simulink model "Doble_pendulo"  (R2024a)
settings: Solver=VariableStepAuto  StartTime=0.0  StopTime=10.0  RelTol=1e-3
values from neighbouring files (symbols this model uses):
  g = 9.81    [exp1.m]
  l1 = 0.3    [exp1.m]
  l2 = 0.25    [exp1.m]
  m1 = 0.2    [exp1.m]
  m2 = 0.1    [exp1.m]
settings Model: Creator=Braulio Ramíreza  LastModifiedBy=Braulio Ramíreza

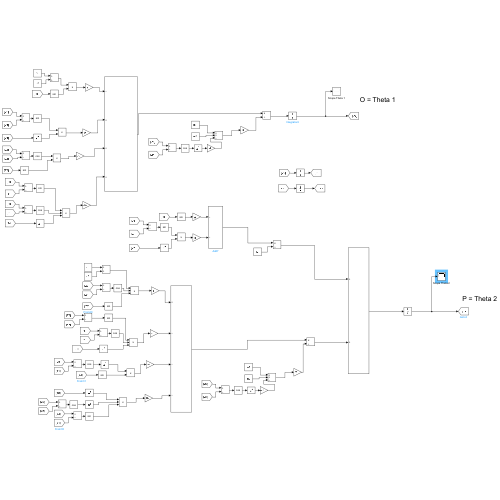
[thumbnail: Simulink's stored preview of the top-level diagram]
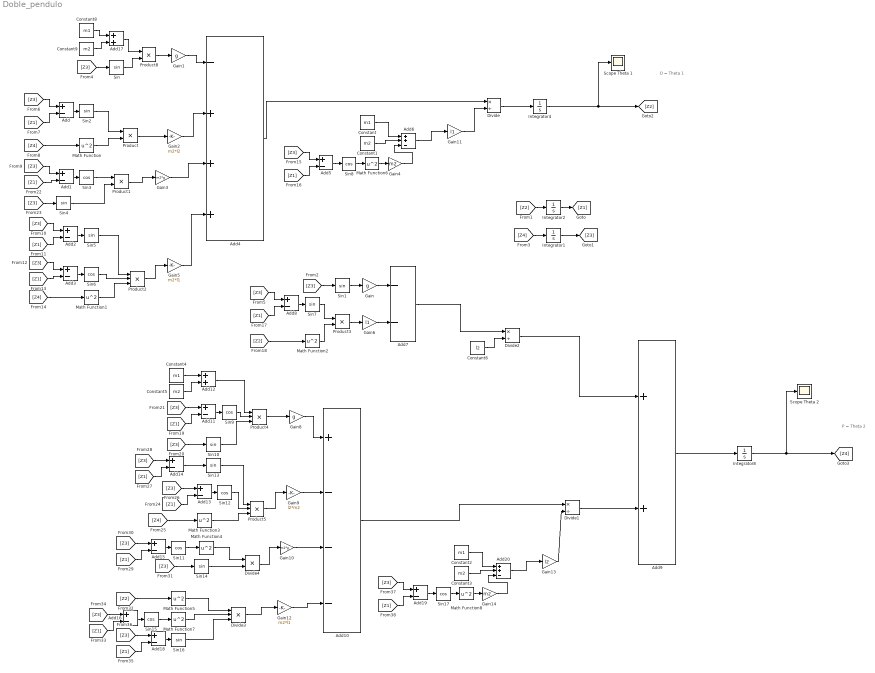
== system Doble_pendulo ==
  note: P = Theta 2
  note: O = Theta 1
  Add{,1..3,5,8,11,13..16,18..19} (13 alike) : Sum  Inputs=+-
  Add10 : Sum  Inputs=+---
  Add12 : Sum
  Add17 : Sum
  Add20 : Sum  Inputs=++-
  Add4 : Sum  Inputs=-+++
  Add6 : Sum  Inputs=++-
  Add7 : Sum  Inputs=--
  Add9 : Sum
  Constant{,2,4,8} (4 alike) : Constant  Value=m1
  Constant{1,3,5,9} (4 alike) : Constant  Value=m2
  Constant6 : Constant  Value=l2
  Divide : Product  Inputs=*/
  Divide1 : Product  Inputs=*/
  Divide2 : Product  Inputs=*/
  Divide3 : Product  Inputs=***
  Divide4 : Product  Inputs=**
  Gain : Gain  Gain=g
  Gain1 : Gain  Gain=g
  Gain10 : Gain  Gain=m2*g
  Gain11 : Gain  Gain=l1
  Gain12 : Gain  Gain=m2*l1
  Gain13 : Gain  Gain=l2
  Gain14 : Gain  Gain=m2
  Gain2 : Gain  Gain=m2*l2
  Gain3 : Gain  Gain=m2*g
  Gain4 : Gain  Gain=m2
  Gain5 : Gain  Gain=m2*l1
  Gain6 : Gain  Gain=l1
  Gain8 : Gain  Gain=g
  Gain9 : Gain  Gain=l2*m2
  Integrator1 : Integrator
  Integrator2 : Integrator
  Integrator4 : Integrator
  Integrator8 : Integrator  InitialCondition=(35*pi)/180
  Math Function{,1..8} (9 alike) : Math  Operator=square
  Product{,1,3,8} (4 alike) : Product
  Product2 : Product  Inputs=3
  Product4 : Product  Inputs=3
  Product5 : Product  Inputs=3
  Scope Theta 1 : Scope
  Scope Theta 2 : Scope
  Sin{,1..2,4..5,7,10,13..14,16} (10 alike) : Trigonometry
  Sin{3,6,8..9,11..12,15,17} (8 alike) : Trigonometry  Operator=cos
  wires:
  [Z2] -> Integrator2/1
  Integrator2/1 -> [Z1]
  Integrator1/1 -> [Z3]
  [Z4] -> Integrator1/1
  Sin15/1 -> Math Function7/1
  Constant4/1 -> Add12/1
  [Z1] -> Add15/2
  Sin/1 -> Product8/2
  Add19/1 -> Sin17/1
  Add13/1 -> Sin12/1
  Add10/1 -> Divide1/1
  Gain/1 -> Add7/1
  [Z1] -> Add3/2
  Math Function8/1 -> Gain14/1
  Constant3/1 -> Add20/2
  Divide3/1 -> Gain12/1
  Gain1/1 -> Add4/1
  [Z1] -> Add5/2
  [Z1] -> Add2/2
  Math Function4/1 -> Divide4/1
  Gain5/1 -> Add4/4
  Sin17/1 -> Math Function8/1
  Add20/1 -> Gain13/1
  [Z3] -> Add19/1
  [Z3] -> Add14/1
  Gain12/1 -> Add10/4
  Add2/1 -> Sin5/1
  Math Function5/1 -> Divide3/1
  Divide4/1 -> Gain10/1
  [Z2] -> Math Function5/1
  [Z3] -> Add15/1
  [Z3] -> Add16/1
  Add15/1 -> Sin11/1
  Product3/1 -> Gain6/1
  Add1/1 -> Sin3/1
  [Z3] -> Add/1
  Constant5/1 -> Add12/2
  Constant8/1 -> Add17/1
  Math Function3/1 -> Product5/3
  [Z1] -> Add18/2
  [Z1] -> Add/2
  Constant9/1 -> Add17/2
  [Z1] -> Add14/2
  Add12/1 -> Product4/1
  Add14/1 -> Sin13/1
  [Z1] -> Add8/2
  Divide/1 -> Integrator4/1
  [Z3] -> Add5/1
  Sin13/1 -> Product5/1
  Sin12/1 -> Product5/2
  [Z3] -> Sin10/1
  [Z3] -> Add13/1
  [Z1] -> Add13/2
  Sin9/1 -> Product4/2
  Gain2/1 -> Add4/2
  Sin11/1 -> Math Function4/1
  [Z3] -> Add11/1
  Add8/1 -> Sin7/1
  [Z3] -> Sin14/1
  [Z2] -> Math Function2/1
  Gain6/1 -> Add7/2
  Sin1/1 -> Gain/1
  Math Function2/1 -> Product3/2
  Add17/1 -> Product8/1
  Sin5/1 -> Product2/1
  Sin4/1 -> Product1/2
  Product8/1 -> Gain1/1
  Add11/1 -> Sin9/1
  Add/1 -> Sin2/1
  Math Function1/1 -> Product2/3
  Add3/1 -> Sin6/1
  Product5/1 -> Gain9/1
  Add6/1 -> Gain11/1
  Product2/1 -> Gain5/1
  Add4/1 -> Divide/1
  [Z1] -> Add11/2
  [Z4] -> Math Function1/1
  Sin8/1 -> Math Function6/1
  Gain4/1 -> Add6/3
  [Z3] -> Add3/1
  [Z3] -> Add2/1
  Math Function6/1 -> Gain4/1
  [Z1] -> Add1/2
  Sin2/1 -> Product/1
  Gain3/1 -> Add4/3
  Product1/1 -> Gain3/1
  Math Function/1 -> Product/2
  Product/1 -> Gain2/1
  [Z3] -> Sin/1
  Add9/1 -> Integrator8/1
  Constant1/1 -> Add6/2
  [Z3] -> Add8/1
  Sin16/1 -> Divide3/3
  [Z3] -> Sin1/1
  Gain8/1 -> Add10/1
  Sin14/1 -> Divide4/2
  [Z3] -> Add1/1
  Integrator4/1 -> Scope Theta 1/1, [Z2]
  [Z4] -> Math Function3/1
  Integrator8/1 -> Scope Theta 2/1, [Z4]
  Sin10/1 -> Product4/3
  Constant2/1 -> Add20/1
  [Z3] -> Sin4/1
  Gain10/1 -> Add10/3
  Add5/1 -> Sin8/1
  Sin3/1 -> Product1/1
  Constant/1 -> Add6/1
  Math Function7/1 -> Divide3/2
  [Z4] -> Math Function/1
  Add16/1 -> Sin15/1
  Add7/1 -> Divide2/1
  Add18/1 -> Sin16/1
  [Z3] -> Add18/1
  Constant6/1 -> Divide2/2
  Gain9/1 -> Add10/2
  Product4/1 -> Gain8/1
  Gain14/1 -> Add20/3
  Sin6/1 -> Product2/2
  Gain13/1 -> Divide1/2
  Divide1/1 -> Add9/2
  Sin7/1 -> Product3/1
  Divide2/1 -> Add9/1
  Gain11/1 -> Divide/2
  [Z1] -> Add16/2
  [Z1] -> Add19/2
